simulink model "pendulum_model"  (R2025b)
settings: Solver=ode45  StartTime=0.0  StopTime=10.0  MaxStep=dtMax  RelTol=1e-3
undefined symbols (not defined in the file): b, g, L, m, theta0, thetaDot0
settings Model: Creator=nuris  LastModifiedBy=nuris
settings DataIOCC: SignalLogging=off  ReturnWorkspaceOutputs=off

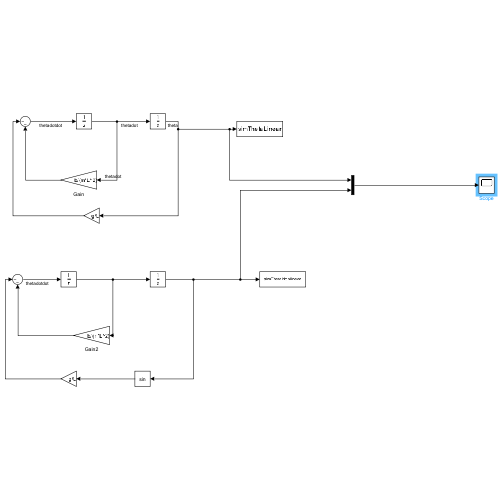
[thumbnail: Simulink's stored preview of the top-level diagram]
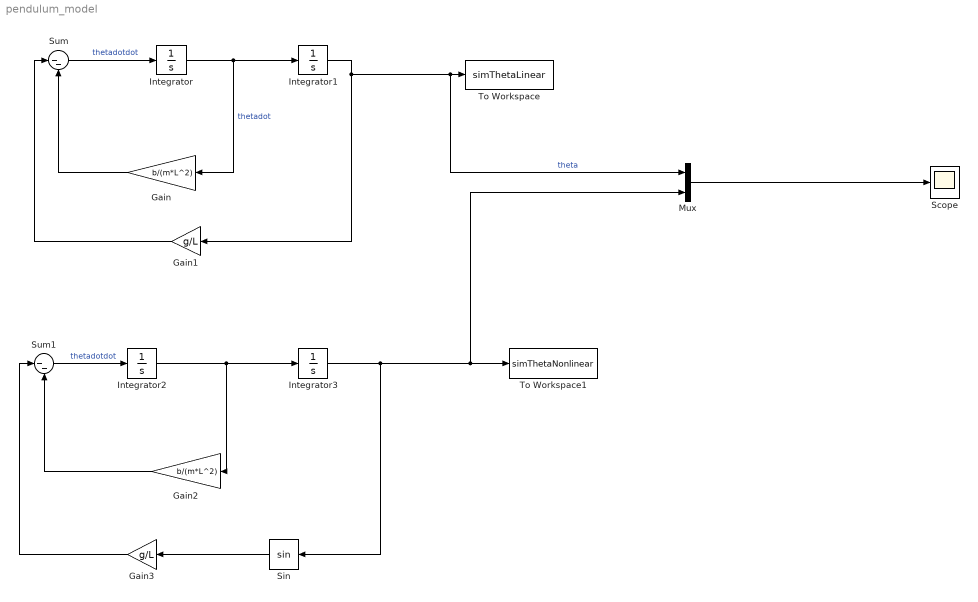
== system pendulum_model ==
  Gain : Gain  Gain=b/(m*L^2)
  Gain1 : Gain  Gain=g/L
  Gain2 : Gain  Gain=b/(m*L^2)
  Gain3 : Gain  Gain=g/L
  Integrator : Integrator  InitialCondition=thetaDot0
  Integrator1 : Integrator  InitialCondition=theta0
  Integrator2 : Integrator  InitialCondition=thetaDot0
  Integrator3 : Integrator  InitialCondition=theta0
  Mux : Mux  Inputs=2
  Scope : Scope
      settings: ActiveDisplayYMinimum=-3.6511766232173253  ActiveDisplayYMaximum=4.0902702679010652
  Sin : Trigonometry
  Sum : Sum  Inputs=|--
  Sum1 : Sum  Inputs=|--
  To Workspace : ToWorkspace  VariableName=simThetaLinear  SaveFormat=Structure With Time  SampleTime=-1
  To Workspace1 : ToWorkspace  VariableName=simThetaNonlinear  SaveFormat=Structure With Time  SampleTime=-1
  wires:
  Integrator/1 -> Gain/1, Integrator1/1  "thetadot"
  Integrator1/1 -> Mux/1, To Workspace/1, Gain1/1  "theta"
  Sum/1 -> Integrator/1  "thetadotdot"
  Gain/1 -> Sum/2
  Gain1/1 -> Sum/1
  Integrator2/1 -> Gain2/1, Integrator3/1
  Gain2/1 -> Sum1/2
  Sum1/1 -> Integrator2/1  "thetadotdot"
  Integrator3/1 -> Sin/1, Mux/2, To Workspace1/1
  Sin/1 -> Gain3/1
  Gain3/1 -> Sum1/1
  Mux/1 -> Scope/1
